simulink model "reaction_pendulum_combined"  (R2021b)
settings: Solver=FixedStepDiscrete  StartTime=0.0  StopTime=30  FixedStep=h  RelTol=1e-3  EnableMultiTasking=on
PreLoadFcn:
  | warning('off','MATLAB:dispatcher:InexactMatch');
InitFcn:
  | startup_sequence
StartFcn:
  | startup_sequence
model workspace (MAT data in the model file):
  square_freq = 0.5
values from neighbouring files (symbols this model uses):
  h = 0.05    [hwinit.m]
  K_LQR = lqr(A,B,Q,R)    [LQR_gain.m]
  linearization_point = [0;0;0]    [startup_sequence.m]
  lp_deviation = [pi/9;0;0]    [startup_sequence.m]
  T = 0:h:T_f    [combi_input_signal.m]
undefined symbols (not defined in the file or in its folder): A_MPC_con, b_MPC_con, dim, gains, H_nlobs, M_MPC, P_MPC, Q_MPC, R_MPC, S
libraries: simulink x1
settings Model: ExtModeTrigDuration=100000  Creator=user  LastModifiedBy=niels
settings DataIOCC: SaveFormat=Array  SignalLoggingSaveFormat=ModelDataLogs  SaveOutput=off  SignalLogging=off  DSMLogging=off  SaveTime=off  ReturnWorkspaceOutputs=off
settings OptimizationCC: ExpressionDepthLimit=2147483647  LifeSpan=inf
settings DebuggingCC: UnderspecifiedInitializationDetection=Classic  MergeDetectMultiDrivingBlocksExec=none  SolverPrmCheckMsg=warning  FcnCallInpInsideContextMsg=warning  StateNameClashWarn=warning  SFUnexpectedBacktrackingDiag=warning  SFNoUnconditionalDefaultTransitionDiag=warning  SFExecutionAtInitializationDiag=none  ArithmeticOperatorsInVariantConditions=warning
settings HardwareCC: ProdBitPerPointer=32  ProdBitPerSizeT=32  ProdBitPerPtrDiffT=32  ProdLargestAtomicFloat=None  ProdIntDivRoundTo=Undefined  ProdEndianess=Unspecified  ProdWordSize=32  ProdHWDeviceType=32-bit Generic
settings ModelReferenceCC: PropagateSignalLabelsOutOfModel=off
settings SFSimCC: SimUseLocalCustomCode=off  CustomCodeUndefinedFunction=UseInterfaceOnly
settings RTWCC: Description=rpend RTDAC/USB2 (Visual C/C++)  SystemTargetFile=rtcon_rpend_usb2.tlc  TemplateMakefile=rtcon_rpend_vc_usb2_x64.tmf  RTWUseLocalCustomCode=off
settings CodeAppCC: StateflowObjectComments=on
settings STFCustomTargetCC: ModelReferenceCompliant=off  CombineOutputUpdateFcns=on  MatFileLogging=on  GRTInterface=off  SystemTargetFile=rtcon_rpend_usb2.tlc
settings GRTTargetCC: TargetLangStandard=C89/C90 (ANSI)  ModelReferenceCompliant=off  ParMdlRefBuildCompliant=off  CompOptLevelCompliant=off  ConcurrentExecutionCompliant=off  CPPClassGenCompliant=off  UseToolchainInfoCompliant=off  ExtMode=on  ExtModeMexFile=rtcon_ext_comm
settings ConfigComp: CovMetricSettings=dw  CovSaveCumulativeToWorkspaceVar=on  CovSaveSingleToWorkspaceVar=on  CovExternalEMLEnable=off  CovSFcnEnable=off

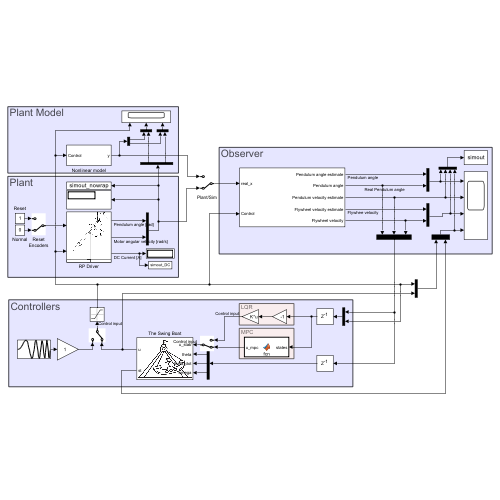
[thumbnail: Simulink's stored preview of the top-level diagram]
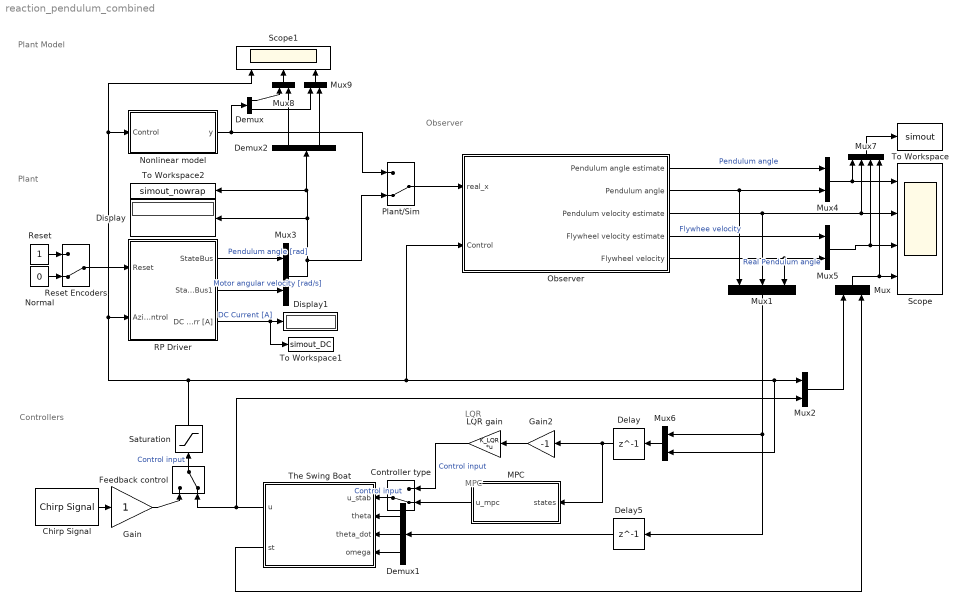
== system reaction_pendulum_combined ==
  note: MPC
  note: LQR
  note: Plant Model
  note: Controllers
  note: Observer
  note: Plant
  Chirp Signal : simulink/Sources/Chirp Signal  f1=0.1  T=30  f2=1
  Controller type : ManualSwitch  CurrentSetting=0
  Delay : Delay  DelayLength=1
  Delay5 : Delay  DelayLength=1
  Demux : Demux  Outputs=2
  Demux1 : Demux  Outputs=3
  Demux2 : Demux  Outputs=2
  Display : Display
  Display1 : Display
  Feedback control : ManualSwitch  CurrentSetting=0
  Gain : Gain
  Gain2 : Gain  Gain=-1
  LQR gain : Gain  Gain=K_LQR  Multiplication=Matrix(K*u)
  MPC : MATLAB Function  TreatAsAtomicUnit=on
  Mux{,2..6,8..9} (8 alike) : Mux  Inputs=2
  Mux1 : Mux  Inputs=3
  Mux7 : Mux
  Nonlinear model : Subsystem
  Normal : Constant  Value=0
  Observer : Subsystem
  Plant/Sim : ManualSwitch  CurrentSetting=0
  RP Driver : Subsystem
      mask Display: image('$imagefile'); % Use "Edit Image" on toolstrip to change.
  Reset : Constant
  Reset Encoders : ManualSwitch  CurrentSetting=0
  Saturation : Saturate  UpperLimit=1  LowerLimit=-1
  Scope : Scope  NumInputPorts=4
  Scope1 : Scope  NumInputPorts=3
  The Swing Boat : Stateflow chart  TreatAsAtomicUnit=on
  To Workspace : ToWorkspace  VariableName=simout  SaveFormat=Structure With Time  SampleTime=-1
  To Workspace1 : ToWorkspace  VariableName=simout_DC  SaveFormat=Structure With Time  SampleTime=-1
  To Workspace2 : ToWorkspace  VariableName=simout_nowrap  SaveFormat=Structure With Time  SampleTime=-1
  wires:
  Normal/1 -> Reset Encoders/2
  Reset/1 -> Reset Encoders/1
  Reset Encoders/1 -> RP Driver/1(Reset)
  RP Driver/1(StateBus) -> Mux3/1  "Pendulum angle [rad]"
  Mux4/1 -> Scope/1, Mux7/1
  Mux5/1 -> Scope/3, Mux7/3
  RP Driver/2(StateBus1) -> Mux3/2  "Motor angular velocity [rad/s]"
  Observer/3(Pendulum velocity estimate) -> Scope/2, Mux7/2, Mux1/2
  Observer/4(Flywheel velocity estimate) -> Mux5/1  "Flywhee velocity"
  Observer/5(Flywheel velocity) -> Mux1/3, Mux5/2
  Mux3/1 -> Plant/Sim/2, Demux2/1, To Workspace2/1, Display/1
  Demux1/2 -> The Swing Boat/3(theta_dot)
  Demux1/3 -> The Swing Boat/4(omega)
  Demux1/1 -> The Swing Boat/2(theta)
  Observer/1(Pendulum angle estimate) -> Mux4/1  "Pendulum angle"
  Observer/2(Pendulum angle) -> Mux1/1, Mux4/2  "Real Pendulum angle"
  Mux/1 -> Scope/4, Mux7/4
  Delay5/1 -> Demux1/1
  Gain2/1 -> LQR gain/1
  Controller type/1 -> The Swing Boat/1(u_stab)  "Control input"
  Mux1/1 -> Delay5/1, Mux6/1
  MPC/1(u_mpc) -> Controller type/2
  LQR gain/1 -> Controller type/1  "Control input"
  The Swing Boat/1(u) -> Mux2/2, Feedback control/2
  The Swing Boat/2(st) -> Mux/2
  RP Driver/3(DC Curr [A]) -> To Workspace1/1, Display1/1  "DC Current [A]"
  Mux2/1 -> Mux/1
  Saturation/1 -> Scope1/1, Nonlinear model/1(Control), RP Driver/2(Azimuth Control), Observer/2(Control), Mux6/2, Mux2/1
  Mux6/1 -> Delay/1
  Delay/1 -> MPC/1(states), Gain2/1
  Mux7/1 -> To Workspace/1
  Chirp Signal/1 -> Gain/1
  Gain/1 -> Feedback control/1
  Feedback control/1 -> Saturation/1  "Control input"
  Nonlinear model/1(y) -> Demux/1, Plant/Sim/1
  Plant/Sim/1 -> Observer/1(real_x)
  Mux8/1 -> Scope1/2
  Mux9/1 -> Scope1/3
  Demux2/2 -> Mux9/2
  Demux/2 -> Mux9/1
  Demux2/1 -> Mux8/2
  Demux/1 -> Mux8/1

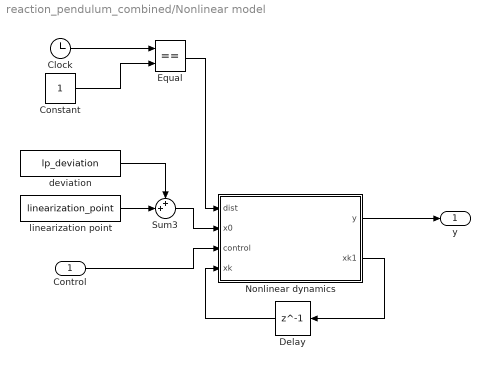
== system reaction_pendulum_combined/Nonlinear model ==
  Control : Inport
  Clock : Clock
  Constant : Constant
  Delay : Delay  DelayLength=1
  Equal : RelationalOperator  Operator===  OutDataTypeStr=boolean  RndMeth=Simplest
  Nonlinear dynamics : MATLAB Function  TreatAsAtomicUnit=on
  Sum3 : Sum  Inputs=++|
  deviation : Constant  Value=lp_deviation
  linearization point : Constant  Value=linearization_point
  y : Outport
  wires:
  Delay/1 -> Nonlinear dynamics/4(xk)
  Sum3/1 -> Nonlinear dynamics/2(x0)
  Control/1 -> Nonlinear dynamics/3(control)
  Nonlinear dynamics/2(xk1) -> Delay/1
  Nonlinear dynamics/1(y) -> y/1
  deviation/1 -> Sum3/1
  linearization point/1 -> Sum3/2
  Clock/1 -> Equal/1
  Constant/1 -> Equal/2
  Equal/1 -> Nonlinear dynamics/1(dist)

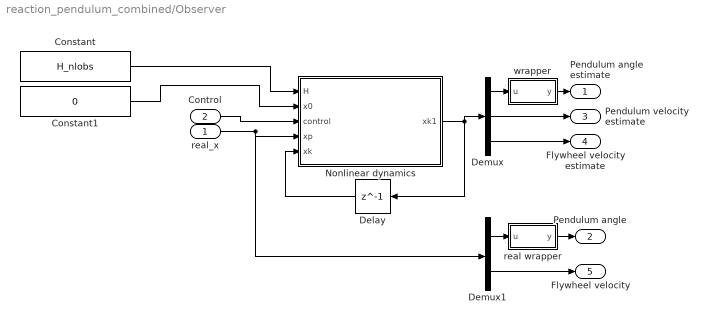
== system reaction_pendulum_combined/Observer ==
  real_x : Inport
  Control : Inport  Port=2
  Constant : Constant  Value=H_nlobs
  Constant1 : Constant  Value=0
  Delay : Delay  DelayLength=1
  Demux : Demux  Outputs=3
  Demux1 : Demux  Outputs=2
  Nonlinear dynamics : MATLAB Function  TreatAsAtomicUnit=on
  real wrapper : MATLAB Function  TreatAsAtomicUnit=on
  wrapper : MATLAB Function  TreatAsAtomicUnit=on
  Pendulum angle estimate : Outport
  Pendulum angle : Outport  Port=2
  Pendulum velocity estimate : Outport  Port=3
  Flywheel velocity estimate : Outport  Port=4
  Flywheel velocity : Outport  Port=5
  wires:
  Delay/1 -> Nonlinear dynamics/5(xk)
  Control/1 -> Nonlinear dynamics/3(control)
  Nonlinear dynamics/1(xk1) -> Demux/1, Delay/1
  real_x/1 -> Demux1/1, Nonlinear dynamics/4(xp)
  Constant/1 -> Nonlinear dynamics/1(H)
  Constant1/1 -> Nonlinear dynamics/2(x0)
  Demux/2 -> Pendulum velocity estimate/1
  Demux/3 -> Flywheel velocity estimate/1
  Demux1/2 -> Flywheel velocity/1
  Demux/1 -> wrapper/1(u)
  wrapper/1(y) -> Pendulum angle estimate/1
  Demux1/1 -> real wrapper/1(u)
  real wrapper/1(y) -> Pendulum angle/1

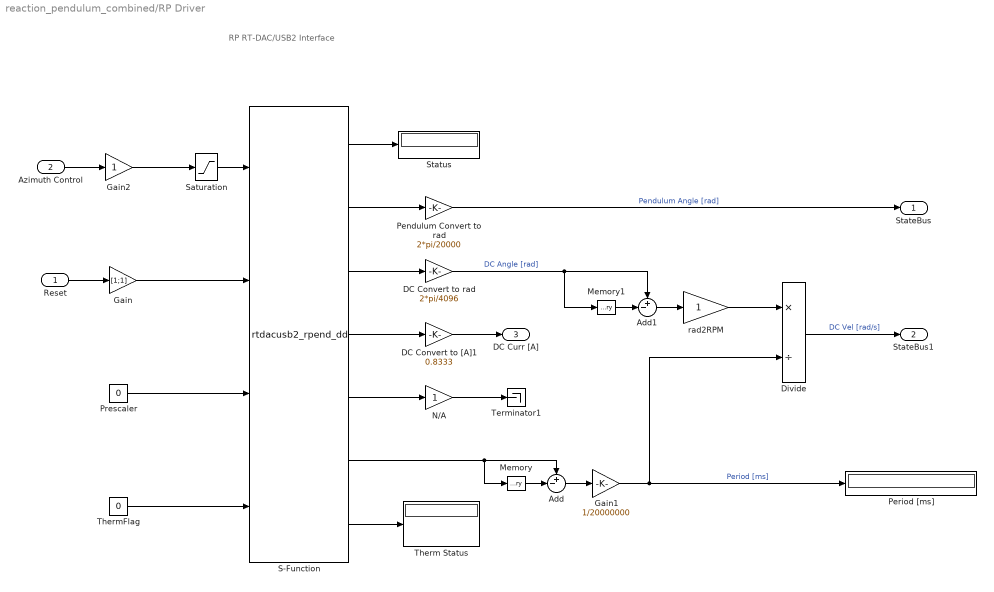
== system reaction_pendulum_combined/RP Driver ==
  note: RP RT-DAC/USB2
      | Interface
  Reset : Inport
  Azimuth Control : Inport  Port=2
  Add : Sum  Inputs=+-|
  Add1 : Sum  Inputs=+-|
  DC Convert to [A]1 : Gain  Gain=0.8333  SaturateOnIntegerOverflow=on  OutDataTypeStr=Inherit: Same as input  ParamDataTypeStr=Inherit: Same as input
  DC Convert to rad : Gain  Gain=2*pi/4096  SaturateOnIntegerOverflow=on  OutDataTypeStr=Inherit: Same as input  ParamDataTypeStr=Inherit: Same as input
  Divide : Product  Inputs=*/
  Gain : Gain  Gain=[1;1]
  Gain1 : Gain  Gain=1/20000000
  Gain2 : Gain
  Memory : Memory
  Memory1 : Memory
  N/A : Gain  SaturateOnIntegerOverflow=on  OutDataTypeStr=Inherit: Same as input  ParamDataTypeStr=Inherit: Same as input
  Pendulum Convert to rad : Gain  Gain=2*pi/20000  SaturateOnIntegerOverflow=on  OutDataTypeStr=Inherit: Same as input  ParamDataTypeStr=Inherit: Same as input
  Period [ms] : Display
  Prescaler : Constant  Value=0
  S-Function : S-Function  FunctionName=rtdacusb2_rpend_dd  Parameters=1, h  SFunctionDeploymentMode=off  EnableBusSupport=off
  Saturation : Saturate  UpperLimit=1  LowerLimit=-1
  Status : Display
  Terminator1 : Terminator
  Therm Status : Display
  ThermFlag : Constant  Value=0
  rad2RPM : Gain  SaturateOnIntegerOverflow=on  OutDataTypeStr=Inherit: Same as input  ParamDataTypeStr=Inherit: Same as input
  StateBus : Outport  VectorParamsAs1DForOutWhenUnconnected=off
  StateBus1 : Outport  Port=2  VectorParamsAs1DForOutWhenUnconnected=off
  DC Curr [A] : Outport  Port=3  VectorParamsAs1DForOutWhenUnconnected=off
  wires:
  S-Function/7 -> Therm Status/1
  S-Function/5 -> N/A/1
  S-Function/4 -> DC Convert to [A]1/1
  ThermFlag/1 -> S-Function/4
  Prescaler/1 -> S-Function/3
  Gain/1 -> S-Function/2
  DC Convert to [A]1/1 -> DC Curr [A]/1
  Divide/1 -> StateBus1/1  "DC Vel [rad/s]"
  rad2RPM/1 -> Divide/1
  Add1/1 -> rad2RPM/1
  Memory1/1 -> Add1/2
  N/A/1 -> Terminator1/1
  S-Function/6 -> Add/1, Memory/1
  Gain2/1 -> Saturation/1
  Gain1/1 -> Period [ms]/1, Divide/2  "Period [ms]"
  Add/1 -> Gain1/1
  Memory/1 -> Add/2
  DC Convert to rad/1 -> Add1/1, Memory1/1  "DC Angle [rad]"
  S-Function/3 -> DC Convert to rad/1
  Pendulum Convert to rad/1 -> StateBus/1  "Pendulum Angle [rad]"
  S-Function/2 -> Pendulum Convert to rad/1
  S-Function/1 -> Status/1
  Saturation/1 -> S-Function/1
  Reset/1 -> Gain/1
  Azimuth Control/1 -> Gain2/1

== stateflow chart reaction_pendulum_combined/The Swing Boat ==
  state Swing_up
    u=-ku*sign(theta_dot);
    st = -0.1;
  state Nothing
    u=0;
    st = 0;
  state Slow_down
    u=kp*sign(theta_dot);
    st = 0.1;
  state Stabilizing
    u=u_stab;
    st=0.4;
  state Flywheel_limit
    u=0;
  Nothing -> Swing_up [order 1] : [abs(theta)>wheel]
  Swing_up -> Nothing : [abs(theta)<wheel]
  Nothing -> Slow_down [order 3] : [abs(theta)<pi/2 && abs(theta_dot)>vmax]
  Slow_down -> Nothing : [abs(theta_dot)<3/4*vmax]
  Nothing -> Stabilizing [order 2] : [abs(theta) < delta]
  Stabilizing -> Nothing [order 1] : [abs(theta) > delta]
  (default) -> Nothing
  Flywheel_limit -> Stabilizing : [abs(omega)<200]
  Stabilizing -> Flywheel_limit [order 2] : [abs(omega)>250]
  data: u_stab input; theta input; theta_dot input; u output; ku local =0.8; kp local =1; delta local =deg2rad(20); vmax local =6; wheel local =pi-deg2rad(60); st output; omega input

== matlab function reaction_pendulum_combined/Observer/wrapper ==
  data: u input; y output
function y = fcn(u)

y = mod(u,2*pi)-pi;

end

== matlab function reaction_pendulum_combined/Observer/real wrapper ==
  data: u input; y output
function y = fcn(u)

y = mod(u,2*pi)-pi;

end

== matlab function reaction_pendulum_combined/MPC ==
  data: states input; u_mpc output; T parameter; S parameter; Q_MPC parameter; R_MPC parameter; dim parameter; P_MPC parameter; M_MPC parameter; A_MPC_con parameter; b_MPC_con parameter
function u_mpc = fcn(states, T,S,Q_MPC,R_MPC,dim,P_MPC,M_MPC,A_MPC_con, b_MPC_con)
    x0 = states;
    [left,right]=costgen(T,S,Q_MPC,R_MPC,dim,x0,P_MPC,M_MPC);
    u0 = zeros(size(right));
%     u_mpc = 0;
    opts = optimoptions('quadprog','Display','off','Algorithm','active-set');
    u_N = quadprog(left,right,A_MPC_con,b_MPC_con,[],[],[],[],u0,opts);
    u_mpc = u_N(1);
end

function [H,h]=costgen(T,S,Q,R,dim,x0,P,M)
    % Cost function generation
    % Converts a cost function of the form:
    % V_N(x(0),u_n) = 0.5*sum_{0,N-1}(x'Qx + u'Ru + 2x'Mu) + 0.5x_N'Px_N
    % into a form only dependent on u_N:
    % V_N(u_N) = 0.5u'Hu + h'u + c
    
    if nargin == 6
        M = zeros(dim.nx,dim.nu);
        P = Q;
    end
    
    % Define the bar matrices Qbar, Rbar, Mbar
    Qbar = blkdiag(kron(eye(dim.N),Q),P); 
    Rbar = kron(eye(dim.N),R);
    Mbar = [kron(eye(dim.N),M);zeros(dim.nx,dim.N*dim.nu)];
    
    % Calculate H,h,c
    H = (Rbar + S'*Qbar*S + 2*S'*Mbar);  
    
    % Stabilizing version
    h = (S'*Qbar*T*x0 + Mbar'*T*x0);
end

== matlab function reaction_pendulum_combined/Observer/Nonlinear dynamics ==
  data: H input; x0 input; control input; xp input; xk input size=[3,1]; xk1 output size=[3,1]; h parameter; gains parameter
function xk1   = nlrk4(H, x0, control, xp, xk, h, gains)
    persistent initialized
    persistent initialized2

    if isempty(initialized)
        xk1 = [xp(1);x0;xp(2)];
        theta_dd = 0;
        initialized = true;
        return;
    end

    if isempty(initialized2)
        xk1 = [xp(1);x0;xp(2)];
        theta_dd = 0;
        initialized2 = true;
        return;
    end

    function dx = nlf(t,x,u,xp,H,gains)
        C = [1,0,0;0,0,1];

        % Define constants
        K1 = gains.K1;
        K2 = gains.K2;
        K3 = gains.K3;
        K4 = gains.K4;
        K5 = gains.K5;
        K6 = gains.K6;
        K_tau = gains.K_tau;
        
        % System equations
        theta = x(1);
        theta_dot = x(2);
        omega = x(3);
        theta_ddot = -K1*sin(theta)-K2*theta_dot-K3*sign(theta_dot)-K_tau*(K4*u-K5*omega-K6*sign(omega));
        omega_dot = K4*u-K5*omega-K6*sign(omega);
        delta = xp-C*x;
        Linear_term = H*(delta);
        NL_term = [theta_dot; theta_ddot; omega_dot] ;
        dx = NL_term + Linear_term;
    end

    function theta_ddot = theta_ddd(t,x,u,xp,H,gains)
        C = [1,0,0;0,0,1];

        % Define constants
        K1 = gains.K1;
        K2 = gains.K2;
        K3 = gains.K3;
        K4 = gains.K4;
        K5 = gains.K5;
        K6 = gains.K6;
        K_tau = gains.K_tau;
        
        % System equations
        theta = x(1);
        theta_dot = x(2);
        omega = x(3);
        theta_ddot = -K1*sin(theta)-K2*theta_dot-K3*sign(theta_dot)-K_tau*(K4*u-K5*omega-K6*sign(omega));
    end

    theta_dd = theta_ddd(0, xk, control, xp, H,gains);

    % Executes one timestep of the RK4 algorithm
    k1 = nlf(0, xk, control, xp, H,gains);
    k2 = nlf(0 + h/2, xk + h/2*k1, control, xp + h/2*k1([1,3]), H,gains);
    k3 = nlf(0 + h/2, xk + h/2*k2, control, xp + h/2*k2([1,3]), H,gains);
    k4 = nlf(0 + h, xk + h*k3, control, xp + h*k3([1,3]), H,gains);
    xk1 = xk + h/6*(k1 + 2*k2 + 2*k3 + k4);

    % % Forward Euler
    % xk1 = xk + h*nlf(0, xk, control);
    % Take out states of interest
    % y = [xk(1); xk(3)];
end

== matlab function reaction_pendulum_combined/Nonlinear model/Nonlinear dynamics ==
  data: dist input; x0 input; y output; control input; xk input size=[3,1]; xk1 output size=[3,1]; h parameter
function [y, xk1] = nlrk4(dist, x0, control, xk, h)
    persistent initialized

    if isempty(initialized)
        xk = x0;
        initialized = true;
    end

    function dx = nlf(t,x,u)
    
        % Define constants
        K1 = 10.6608;
        K2 = 0.0487;
        K3 = 0.1031;
        K4 = 404.3827;
        K5 = 0.9442;
        K6 = 1.7125;
        K_tau = 0.0107;
        
        % System equations
        theta = x(1);
        theta_dot = x(2);
        omega = x(3);
        theta_ddot = -K1*sin(theta)-K2*theta_dot-K3*sign(theta_dot)-K_tau*(K4*u-K5*omega-K6*sign(omega));
        omega_dot = K4*u-K5*omega-K6*sign(omega);
        dx = [theta_dot; theta_ddot; omega_dot];
    end

    % Executes one timestep of the RK4 algorithm
    k1 = nlf(0, xk, control);
    k2 = nlf(0 + h/2, xk + h/2*k1, control);
    k3 = nlf(0 + h/2, xk + h/2*k2, control);
    k4 = nlf(0 + h, xk + h*k3, control);
    xk1 = xk + h/6*(k1 + 2*k2 + 2*k3 + k4);

    % if dist
    %     xk1(1)=pi/9;
    %     xk(1) = pi/9;
    % end

    % % Forward Euler
    % xk1 = xk + h*nlf(0, xk, control);
    % Take out states of interest
    y = [xk(1); xk(3)];
end
